simulink model "test_multiport"  (Simulink 7.5)
settings: Solver=ode45  StartTime=0.0  StopTime=10.0  RelTol=1e-3
values from neighbouring files (symbols this model uses):
  apSampleTime = 0.01    [demoz2SlugsV5.m]
settings Model: Creator=Robert  LastModifiedBy=Robert

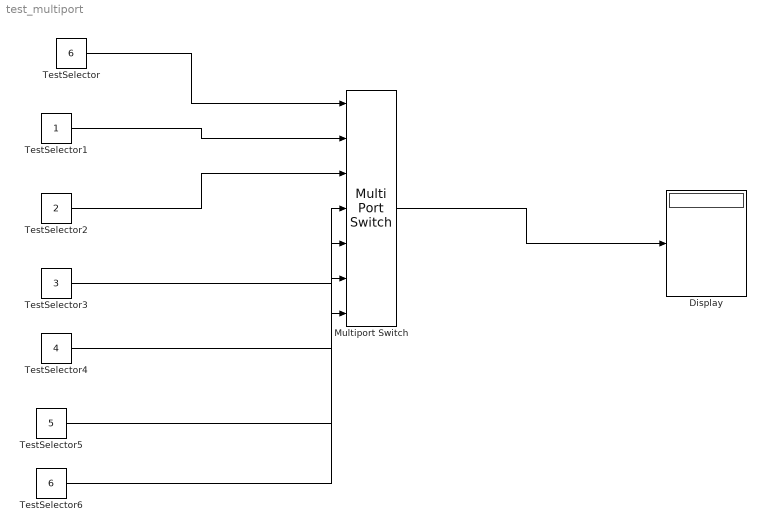
== system test_multiport ==
  Display : Display
  Multiport Switch : MultiPortSwitch  Inputs=6  zeroidx=off  OutDataTypeMode=single  OutDataType=fixdt(1, 16)  OutScaling=2^0  OutDataTypeStr=single  SampleTime=apSampleTime
  TestSelector : Constant  Value=6  OutDataType=fixdt(1, 16)  OutScaling=2^0
  TestSelector1 : Constant  OutDataType=fixdt(1, 16)  OutScaling=2^0
  TestSelector2 : Constant  Value=2  OutDataType=fixdt(1, 16)  OutScaling=2^0
  TestSelector3 : Constant  Value=3  OutDataType=fixdt(1, 16)  OutScaling=2^0
  TestSelector4 : Constant  Value=4  OutDataType=fixdt(1, 16)  OutScaling=2^0
  TestSelector5 : Constant  Value=5  OutDataType=fixdt(1, 16)  OutScaling=2^0
  TestSelector6 : Constant  Value=6  OutDataType=fixdt(1, 16)  OutScaling=2^0
  wires:
  TestSelector/1 -> Multiport Switch/1
  TestSelector1/1 -> Multiport Switch/2
  TestSelector2/1 -> Multiport Switch/3
  TestSelector3/1 -> Multiport Switch/4
  TestSelector4/1 -> Multiport Switch/5
  TestSelector5/1 -> Multiport Switch/6
  TestSelector6/1 -> Multiport Switch/7
  Multiport Switch/1 -> Display/1
